simulink model "lab22"  (Simulink 7.9)
settings: Solver=ode4  StartTime=0.0  StopTime=100.0  FixedStep=0.01  RelTol=1e-3
settings Model: Creator=aziemba  LastModifiedBy=aziemba

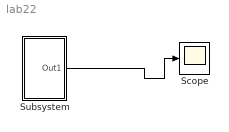
== system lab22 ==
  Scope : Scope
  Subsystem : Subsystem  mask{m=10, k=1, l=3, fi0=90, g=10, t0=0}
      mask prompts: m "masa"; k "wspólczynnik tłumienia"; l "dlugosc liny"; fi0 "kat poczatkowy"; g "grawitacja"; t0 "czas odświerzania"
  wires:
  Subsystem/1(Out1) -> Scope/1

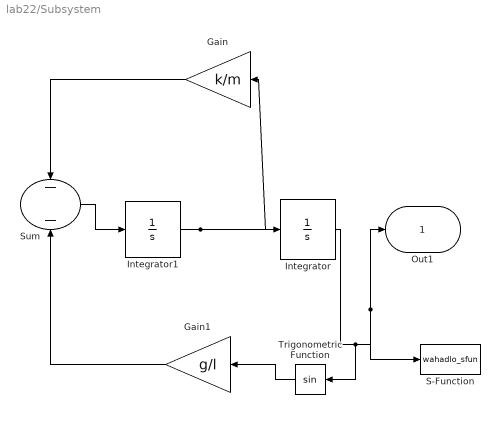
== system lab22/Subsystem ==
  Gain : Gain  Gain=k/m
  Gain1 : Gain  Gain=g/l
  Integrator : Integrator  InitialCondition=(fi0*pi)/180
  Integrator1 : Integrator
  S-Function : S-Function  FunctionName=wahadlo_sfun  Parameters=l,m,fi0,t0  EnableBusSupport=off
  Sum : Sum  Inputs=--
  Trigonometric Function : Trigonometry
  Out1 : Outport
  wires:
  Gain/1 -> Sum/1
  Sum/1 -> Integrator1/1
  Integrator1/1 -> Integrator/1, Gain/1
  Integrator/1 -> Trigonometric Function/1, Out1/1, S-Function/1
  Gain1/1 -> Sum/2
  Trigonometric Function/1 -> Gain1/1
